simulink model "sim_system"  (Simulink 7.9)
settings: Solver=ode45  StartTime=0.0  StopTime=t_sim  RelTol=1e-3
values from neighbouring files (symbols this model uses):
  A_lin = J    [linearisation.m]
  B_lin = [B_lin_Wf B_lin_Ccharge]    [linearisation.m]
  C_charge_0 = f_ctl(Wf_0, Ng_0)    [point_equilibre.m]
  C_lin = [0 1 0 ... (first row only)    [linearisation.m]
  D_lin = [0 0 ... (first row only)    [linearisation.m]
  Ig_norm = ig * (2*pi)/(60*10)    [main.m]
  isong = [20000 21000 22000 23000 24000 25000 26000 27000 28000 29000 30000 31000 ... (16 elements, 16x1)]    [donnees_et_modeles_lineaires.mat]    (also in donnees_turbine_v2007a.mat)
  isowf = [40 80 120 160 200 240 280 320 360 400 440 480 ... (15 elements, 15x1)]    [donnees_et_modeles_lineaires.mat]    (also in donnees_turbine_v2007a.mat)
  Itot_norm = itot *(2*pi)/(60*10)    [main.m]
  Ng_0 = 28000    [point_equilibre.m]
  Ntl_0 = ntlnom    [point_equilibre.m]
  ntlnom = 22800    [donnees_et_modeles_lineaires.mat]    (also in donnees_turbine_v2007a.mat)
  P3_0 = f_p3(Wf_0, Ng_0)    [point_equilibre.m]
  T45_0 = f_t45(Wf_0, Ng_0)    [point_equilibre.m]
  t_sim = 20 ; sim('sim_system_kalman', t_sim)    [main.m]    (also in obs_kalman.m)
  tcg = [-4.72566699982 -2.1958899498 0.325212001801 2.65510463715 5.70554542542 9.11180782318 12.5180749893 15.9243402481 19.3306007385 22.7368736267 26.1431350708 29.5494003296 ... (240 elements, 15x16)]    [donnees_et_modeles_lineaires.mat]    (also in donnees_turbine_v2007a.mat)
  tctl100 = [-0.0806421041489 -0.00261628627777 0.383603572845 0.214125156403 0.554617404938 0.27828836441 0.00195932388306 -0.274368286133 -0.55069732666 -0.827028751373 -1.10335540771 -1.37968444824 ... (240 elements, 15x16)]    [donnees_et_modeles_lineaires.mat]    (also in donnees_turbine_v2007a.mat)
  tdctldntl = [-0.000853070175439 -0.000853070175439 -0.000853070175439 -0.000853070175439 -0.00046798245614 -0.00101842105263 -0.0012701754386 -0.00134210526316 -0.00138728070175 -0.00140219298246 -0.00144561403509 -0.00155526315789 ... (16 elements, 16x1)]    [donnees_et_modeles_lineaires.mat]    (also in donnees_turbine_v2007a.mat)
  tdos = 0.054    [donnees_et_modeles_lineaires.mat]    (also in donnees_turbine_v2007a.mat)
  tp3 = [1.74359560013 1.83476543427 1.89652109146 1.97084283829 2.02915382385 2.07755017281 2.12594628334 2.17434239388 2.22273850441 2.27113461494 2.31953167915 2.36792778969 ... (240 elements, 15x16)]    [donnees_et_modeles_lineaires.mat]    (also in donnees_turbine_v2007a.mat)
  tt4 = [158.323181152 257.927246094 378.081359863 509.409484863 632.046447754 753.55480957 875.063598633 996.572021484 1118.07995605 1239.58874512 1361.09716797 1482.60595703 ... (240 elements, 15x16)]    [donnees_et_modeles_lineaires.mat]    (also in donnees_turbine_v2007a.mat)
  tth = 0.8    [donnees_et_modeles_lineaires.mat]    (also in donnees_turbine_v2007a.mat)
  Wf_0 = fminsearch(@(wf) abs(f_cg(wf,28000)), Wf_init)    [point_equilibre.m]
libraries: simulink_extras x3
settings Model: Creator=maffre  LastModifiedBy=maffre

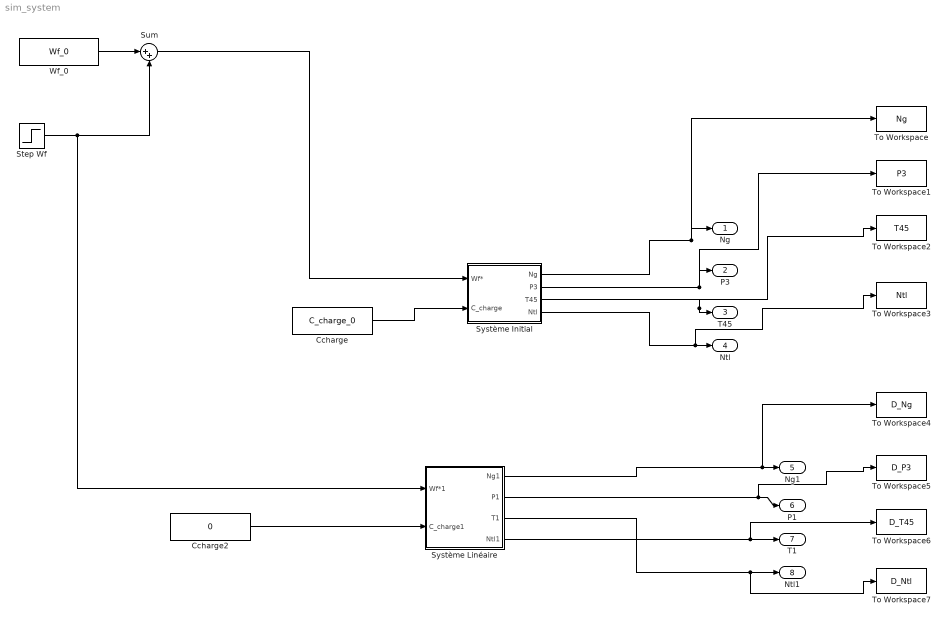
== system sim_system ==
  Ccharge : Constant  Value=C_charge_0
  Ccharge2 : Constant  Value=0
  Step Wf : Step  Time=t_sim/2  After=40  SampleTime=0
  Sum : Sum  Inputs=|++
  Système Initial : Subsystem
  Système Linéaire : Subsystem
  To Workspace : ToWorkspace  VariableName=Ng  SampleTime=-1  SaveFormat=Timeseries
  To Workspace1 : ToWorkspace  VariableName=P3  SampleTime=-1  SaveFormat=Timeseries
  To Workspace2 : ToWorkspace  VariableName=T45  SampleTime=-1  SaveFormat=Timeseries
  To Workspace3 : ToWorkspace  VariableName=Ntl  SampleTime=-1  SaveFormat=Timeseries
  To Workspace4 : ToWorkspace  VariableName=D_Ng  SampleTime=-1  SaveFormat=Timeseries
  To Workspace5 : ToWorkspace  VariableName=D_P3  SampleTime=-1  SaveFormat=Timeseries
  To Workspace6 : ToWorkspace  VariableName=D_T45  SampleTime=-1  SaveFormat=Timeseries
  To Workspace7 : ToWorkspace  VariableName=D_Ntl  SampleTime=-1  SaveFormat=Timeseries
  "Wf_0 " : Constant  Value=Wf_0
  Ng : Outport
  P3 : Outport  Port=2
  T45 : Outport  Port=3
  Ntl : Outport  Port=4
  Ng1 : Outport  Port=5
  P1 : Outport  Port=6
  T1 : Outport  Port=7
  Ntl1 : Outport  Port=8
  wires:
  Système Initial/1(Ng) -> Ng/1, To Workspace/1
  Système Initial/2(P3) -> P3/1, To Workspace1/1
  Système Initial/3(T45) -> T45/1, To Workspace2/1
  Système Initial/4(Ntl) -> Ntl/1, To Workspace3/1
  Système Linéaire/1(Ng1) -> Ng1/1, To Workspace4/1
  Ccharge2/1 -> Système Linéaire/2(C_charge1)
  Système Linéaire/2(P1) -> P1/1, To Workspace5/1
  Système Linéaire/3(T1) -> T1/1, To Workspace6/1
  Système Linéaire/4(Ntl1) -> Ntl1/1, To Workspace7/1
  "Wf_0 "/1 -> Sum/1
  Step Wf/1 -> Sum/2, Système Linéaire/1(Wf*1)
  Sum/1 -> Système Initial/1(Wf*)
  Ccharge/1 -> Système Initial/2(C_charge)

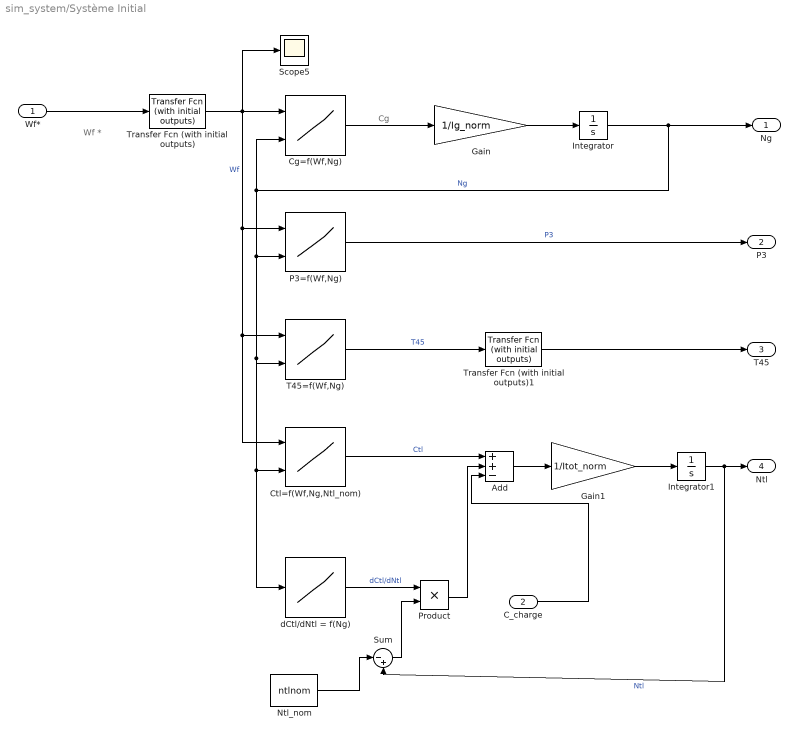
== system sim_system/Système Initial ==
  note: Wf *
  note: Cg
  Wf* : Inport
  C_charge : Inport  Port=2
  Add : Sum  Inputs=++-
  Cg=f(Wf,Ng) : Lookup_n-D  BreakpointsForDimension1=isowf  BreakpointsForDimension2=isong  Table=tcg  RndMeth=Simplest  InputSameDT=on
  Ctl=f(Wf,Ng,Ntl_nom) : Lookup_n-D  BreakpointsForDimension1=isowf  BreakpointsForDimension2=isong  Table=tctl100  RndMeth=Simplest  InputSameDT=on
  Gain : Gain  Gain=1/Ig_norm
  Gain1 : Gain  Gain=1/Itot_norm
  Integrator : Integrator  InitialCondition=Ng_0
  Integrator1 : Integrator  InitialCondition=Ntl_0
  Ntl_nom : Constant  Value=ntlnom
  P3=f(Wf,Ng) : Lookup_n-D  BreakpointsForDimension1=isowf  BreakpointsForDimension2=isong  Table=tp3  RndMeth=Simplest  InputSameDT=on
  Product : Product  RndMeth=Zero
  Scope5 : Scope
      settings: SaveName=ScopeData8
  Sum : Sum  Inputs=|-+
  T45=f(Wf,Ng) : Lookup_n-D  BreakpointsForDimension1=isowf  BreakpointsForDimension2=isong  Table=tt4  RndMeth=Simplest  InputSameDT=on
  Transfer Fcn (with initial outputs) : simulink_extras/Additional Linear/Transfer Fcn (with initial outputs)  N=[1]  D="[tdos  1]"  Y0=Wf_0  U0=Wf_0
  Transfer Fcn (with initial outputs)1 : simulink_extras/Additional Linear/Transfer Fcn (with initial outputs)  N=[1]  D="[tth  1]"  Y0=T45_0  U0=T45_0
  dCtl/dNtl = f(Ng) : Lookup_n-D  NumberOfTableDimensions=1  BreakpointsForDimension1=isong  Table=tdctldntl  RndMeth=Simplest  InputSameDT=on
  Ng : Outport
  P3 : Outport  Port=2
  T45 : Outport  Port=3
  Ntl : Outport  Port=4
  wires:
  Wf*/1 -> Transfer Fcn (with initial outputs)/1
  Transfer Fcn (with initial outputs)1/1 -> T45/1
  T45=f(Wf,Ng)/1 -> Transfer Fcn (with initial outputs)1/1  "T45"
  Ntl_nom/1 -> Sum/1
  Add/1 -> Gain1/1
  Integrator1/1 -> Ntl/1, Sum/2  "Ntl"
  Gain1/1 -> Integrator1/1
  Product/1 -> Add/2
  Ctl=f(Wf,Ng,Ntl_nom)/1 -> Add/1  "Ctl"
  Sum/1 -> Product/2
  dCtl/dNtl = f(Ng)/1 -> Product/1  "dCtl/dNtl"
  P3=f(Wf,Ng)/1 -> P3/1  "P3"
  Transfer Fcn (with initial outputs)/1 -> Cg=f(Wf,Ng)/1, P3=f(Wf,Ng)/1, T45=f(Wf,Ng)/1, Ctl=f(Wf,Ng,Ntl_nom)/1, Scope5/1  "Wf"
  Cg=f(Wf,Ng)/1 -> Gain/1
  Gain/1 -> Integrator/1
  Integrator/1 -> Cg=f(Wf,Ng)/2, P3=f(Wf,Ng)/2, T45=f(Wf,Ng)/2, Ctl=f(Wf,Ng,Ntl_nom)/2, dCtl/dNtl = f(Ng)/1, Ng/1  "Ng"
  C_charge/1 -> Add/3

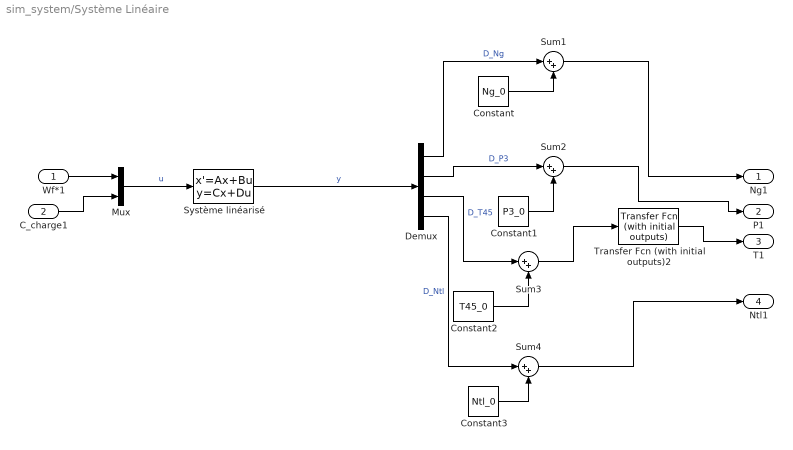
== system sim_system/Système Linéaire ==
  Wf*1 : Inport
  C_charge1 : Inport  Port=2
  Constant : Constant  Value=Ng_0
  Constant1 : Constant  Value=P3_0
  Constant2 : Constant  Value=T45_0
  Constant3 : Constant  Value=Ntl_0
  Demux : Demux
  Mux : Mux  Inputs=2
  Sum{1..4} (4 alike) : Sum  Inputs=|++
  Système linéarisé : StateSpace  A=A_lin  B=B_lin  C=C_lin  D=D_lin
  Transfer Fcn (with initial outputs)2 : simulink_extras/Additional Linear/Transfer Fcn (with initial outputs)  N=[1]  D="[tth  1]"  Y0=T45_0  U0=T45_0
  Ng1 : Outport
  P1 : Outport  Port=2
  T1 : Outport  Port=3
  Ntl1 : Outport  Port=4
  wires:
  Sum4/1 -> Ntl1/1
  Transfer Fcn (with initial outputs)2/1 -> T1/1
  Sum2/1 -> P1/1
  Sum1/1 -> Ng1/1
  Système linéarisé/1 -> Demux/1  "y"
  Mux/1 -> Système linéarisé/1  "u"
  Constant3/1 -> Sum4/2
  Demux/4 -> Sum4/1  "D_Ntl"
  Constant2/1 -> Sum3/2
  Sum3/1 -> Transfer Fcn (with initial outputs)2/1
  Demux/3 -> Sum3/1  "D_T45"
  Constant1/1 -> Sum2/2
  Demux/2 -> Sum2/1  "D_P3"
  Constant/1 -> Sum1/2
  Demux/1 -> Sum1/1  "D_Ng"
  Wf*1/1 -> Mux/1
  C_charge1/1 -> Mux/2
